simulink model "gm_EdgeDetectionAndOverlayHDL"  (R2023a)
settings: Solver=FixedStepDiscrete  StartTime=0.0  StopTime=402*324*10  RelTol=1e-3
PreLoadFcn:
  | thresholdValue = 7;
  | alpha = 0.8;
undefined symbols (not defined in the file or in its folder): gray
libraries: visionhdlio x2, visionanalysis x1, visionhdlanalysis x1, visionhdlutilities x1, dspvision x1
settings Model: ModifiedByFormat=The MathWorks Inc.  SimulationMode=accelerator  Creator=The MathWorks, Inc.  LastModifiedBy=The MathWorks Inc.
settings SolverCC: AlgebraicLoopSolver=TrustRegion  MinimalZcImpactIntegration=on
settings DataIOCC: LimitDataPoints=on  SaveFormat=Array  SaveOutput=off  SaveTime=off  ReturnWorkspaceOutputs=off
settings OptimizationCC: BlockReduction=off  ConditionallyExecuteInputs=off  DefaultParameterBehavior=Inlined  LifeSpan=inf
settings DebuggingCC: AlgebraicLoopMsg=error  SolverPrmCheckMsg=warning  InheritedTsInSrcMsg=none  SingleTaskRateTransMsg=error  ParameterPrecisionLossMsg=none  UnconnectedInputMsg=warning  UnconnectedOutputMsg=warning  UnconnectedLineMsg=warning  AllowSymbolicDim=off  SFUnexpectedBacktrackingDiag=warning  SFNoUnconditionalDefaultTransitionDiag=warning  SFExecutionAtInitializationDiag=none  IntegerSaturationMsg=none  ArithmeticOperatorsInVariantConditions=warning
settings HardwareCC: ProdBitPerPointer=32  ProdBitPerSizeT=32  ProdBitPerPtrDiffT=32  ProdLargestAtomicFloat=None  ProdIntDivRoundTo=Undefined  ProdEndianess=Unspecified  ProdWordSize=32  ProdHWDeviceType=ASIC/FPGA->ASIC/FPGA  ProdEqTarget=off
settings ModelReferenceCC: EnableRefExpFcnMdlSchedulingChecks=on  PropagateSignalLabelsOutOfModel=off
settings SFSimCC: SimUseLocalCustomCode=off  CustomCodeUndefinedFunction=UseInterfaceOnly
settings RTWCC: RTWUseLocalCustomCode=off  DLArmComputeVersion=19.05
settings CodeAppCC: StateflowObjectComments=on
settings GRTTargetCC: TargetLangStandard=C89/C90 (ANSI)
settings ConfigComp: CovMetricSettings=dw  CovSaveCumulativeToWorkspaceVar=on  CovSaveSingleToWorkspaceVar=on  CovExternalEMLEnable=off  CovSFcnEnable=off

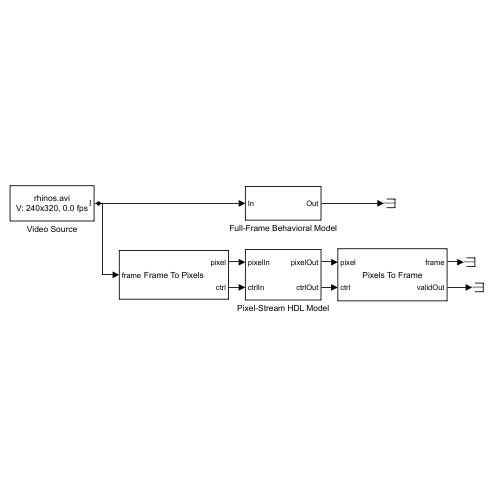
[thumbnail: Simulink's stored preview of the top-level diagram]
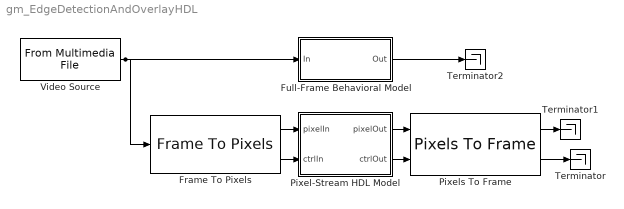
== system gm_EdgeDetectionAndOverlayHDL ==
  Frame To Pixels : visionhdlio/Frame To Pixels  NumComponents=1  NumPixels=1  VideoFormat=240p  ActivePixelsPerLine=320  ActiveVideoLines=240  TotalPixelsPerLine=402  TotalVideoLines=324  StartingActiveLine=1  FrontPorch=44  SampleTime=0  VideoFormatCache=240p  ActivePixelsPerLineCache=32  ActiveVideoLinesCache=18  TotalPixelsPerLineCache=42  TotalVideoLinesCache=28  StartingActiveLineCache=6  FrontPorchCache=5
  Full-Frame Behavioral Model : Subsystem
  Pixel-Stream HDL Model : Subsystem
  Pixels To Frame : visionhdlio/Pixels To Frame  NumComponents=1  NumPixels=1  VideoFormat=240p  ActivePixelsPerLine=320  ActiveVideoLines=240  TotalPixelsPerLine=402  TotalVideoLines=324  VideoFormatCache=240p  ActivePixelsPerLineCache=32  ActiveVideoLinesCache=18  TotalPixelsPerLineCache=42  TotalVideoLinesCache=28
  Terminator : Terminator
  Terminator1 : Terminator
  Terminator2 : Terminator
  Video Source : dspvision/From Multimedia File  inputFilename=rhinos.avi  readRange=[1 Inf]  loop=on  numPlays=inf  outputStreams=Video only  videoDataType=uint8  audioDataType=int16  inheritSampleTime=off  userDefinedSampleTime=402*324  noAudioOutput=off  isIntensityVideo=off  fourcc=Intensity  colorVideoFormat=One multidimensional signal  outputEOF=off  dataOrg=Column-major  audioFrameSize=1024  computeAudioFrameSize=off  outSamplingMode=Sample based
  wires:
  Pixels To Frame/1 -> Terminator1/1
  Pixel-Stream HDL Model/2(ctrlOut) -> Pixels To Frame/2
  Pixel-Stream HDL Model/1(pixelOut) -> Pixels To Frame/1
  Frame To Pixels/2 -> Pixel-Stream HDL Model/2(ctrlIn)
  Frame To Pixels/1 -> Pixel-Stream HDL Model/1(pixelIn)
  Full-Frame Behavioral Model/1(Out) -> Terminator2/1
  Video Source/1 -> Full-Frame Behavioral Model/1(In), Frame To Pixels/1
  Pixels To Frame/2 -> Terminator/1

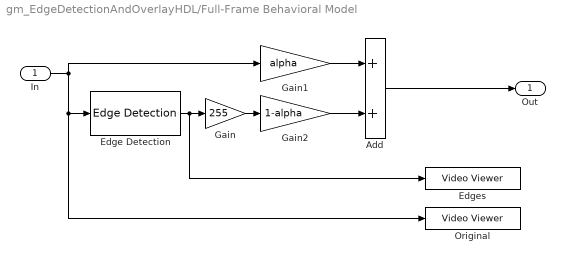
== system gm_EdgeDetectionAndOverlayHDL/Full-Frame Behavioral Model ==
  In : Inport
  Add : Sum  OutDataTypeStr=uint8  SaturateOnIntegerOverflow=on
  Edge Detection : visionanalysis/Edge Detection  method=Sobel  outputType=Binary image  userDefinedThreshold=on  thresholdSource=Specify via dialog  threshold=thresholdValue  thresholdTuning=4  edgeThinning=off  threshold_canny=[0.25 0.60]  autoPercent=70  sigma=1  roundingMode=Floor  overflowMode=on  prodOutputMode=Binary point scaling  prodOutputWordLength=32  prodOutputFracLength=18
  Edges : VideoViewer  colormapValue=gray(256)  FigPos=[454.333333333333 430.666666666667 378 284]
  Gain : Gain  Gain=255  OutDataTypeStr=uint8
  Gain1 : Gain  Gain=alpha  OutDataTypeStr=uint8
  Gain2 : Gain  Gain=1-alpha  OutDataTypeStr=uint8
  Original : VideoViewer  colormapValue=gray(256)  FigPos=[40 427.333333333333 366 282]
  Out : Outport  VectorParamsAs1DForOutWhenUnconnected=off
  wires:
  Add/1 -> Out/1
  In/1 -> Gain1/1, Edge Detection/1, Original/1
  Edge Detection/1 -> Edges/1, Gain/1
  Gain2/1 -> Add/2
  Gain1/1 -> Add/1
  Gain/1 -> Gain2/1

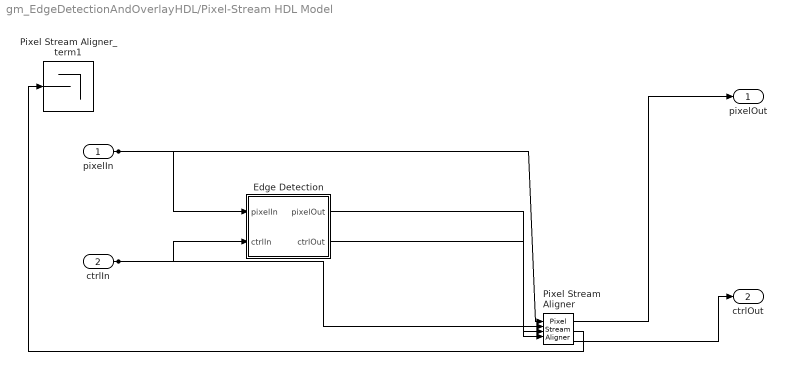
== system gm_EdgeDetectionAndOverlayHDL/Pixel-Stream HDL Model ==
  pixelIn : Inport  OutDataTypeStr=uint8  PortDimensions=1  SampleTime=1
  ctrlIn : Inport  Port=2
  Edge Detection : Subsystem
  Pixel Stream Aligner : visionhdlutilities/Pixel Stream Aligner  LineBufferSize=2048  MaximumNumberOfLines=10  SimulateUsing=Code generation
  Pixel Stream Aligner_term1 : Terminator
  pixelOut : Outport  SampleTime=1  VectorParamsAs1DForOutWhenUnconnected=off
  ctrlOut : Outport  Port=2  VectorParamsAs1DForOutWhenUnconnected=off
  wires:
  pixelIn/1 -> Edge Detection/1(pixelIn), Pixel Stream Aligner/1
  ctrlIn/1 -> Edge Detection/2(ctrlIn), Pixel Stream Aligner/2
  Edge Detection/1(pixelOut) -> Pixel Stream Aligner/3
  Edge Detection/2(ctrlOut) -> Pixel Stream Aligner/4
  Pixel Stream Aligner/1 -> pixelOut/1
  Pixel Stream Aligner/2 -> Pixel Stream Aligner_term1/1
  Pixel Stream Aligner/3 -> ctrlOut/1

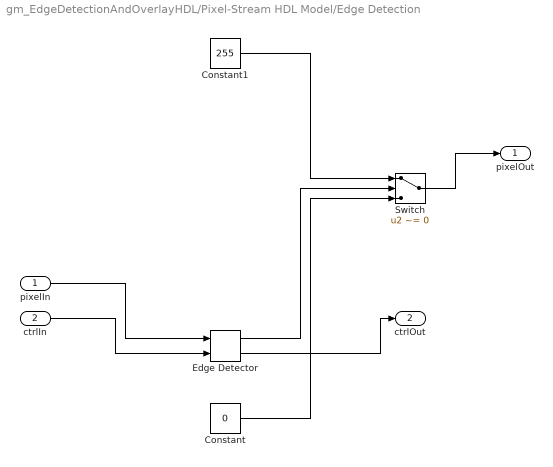
== system gm_EdgeDetectionAndOverlayHDL/Pixel-Stream HDL Model/Edge Detection ==
  pixelIn : Inport  OutDataTypeStr=uint8  PortDimensions=1  SampleTime=1
  ctrlIn : Inport  Port=2
  Constant : Constant  Value=0  OutDataTypeStr=uint8  SampleTime=1
  Constant1 : Constant  Value=255  OutDataTypeStr=uint8  SampleTime=1
  Edge Detector : visionhdlanalysis/Edge Detector  Method=Sobel  BinaryImageOutputPort=on  GradientComponentOutputPorts=off  ThresholdSource=Property  Threshold=thresholdValue  LineBufferSize=2048  PaddingMethod=Symmetric  SimulateUsing=Code generation  roundingMode=Floor  overflowMode=on  GradientMin=[]  GradientMax=[]
  Switch : Switch  Criteria=u2 ~= 0  Threshold=double(0)  OutDataTypeStr=uint8  SampleTime=1  SaturateOnIntegerOverflow=off  InputSameDT=off
  pixelOut : Outport  SampleTime=1  VectorParamsAs1DForOutWhenUnconnected=off
  ctrlOut : Outport  Port=2  VectorParamsAs1DForOutWhenUnconnected=off
  wires:
  pixelIn/1 -> Edge Detector/1
  ctrlIn/1 -> Edge Detector/2
  Constant/1 -> Switch/3
  Constant1/1 -> Switch/1
  Edge Detector/1 -> Switch/2
  Edge Detector/2 -> ctrlOut/1
  Switch/1 -> pixelOut/1
